simulink model "TST_CrCtl_ShOff"  (R2016b)
settings: Solver=FixedStepDiscrete  StartTime=0.0  StopTime=simTime  FixedStep=sampleTime  RelTol=1e-3
values from neighbouring files (symbols this model uses):
  testCase = 1    [initTST_CrCtl_ShOff_001.m]    (also in initTST_CrCtl_ShOff_002.m = 2; initTST_CrCtl_ShOff_003.m = 3)
libraries: simulink x31, UnitTest_Lib x15
(part 1 of 2)
settings Model: Creator=guanxiaoxing  LastModifiedBy=guanxiaoxing
settings DebuggingCC: SignalRangeChecking=error

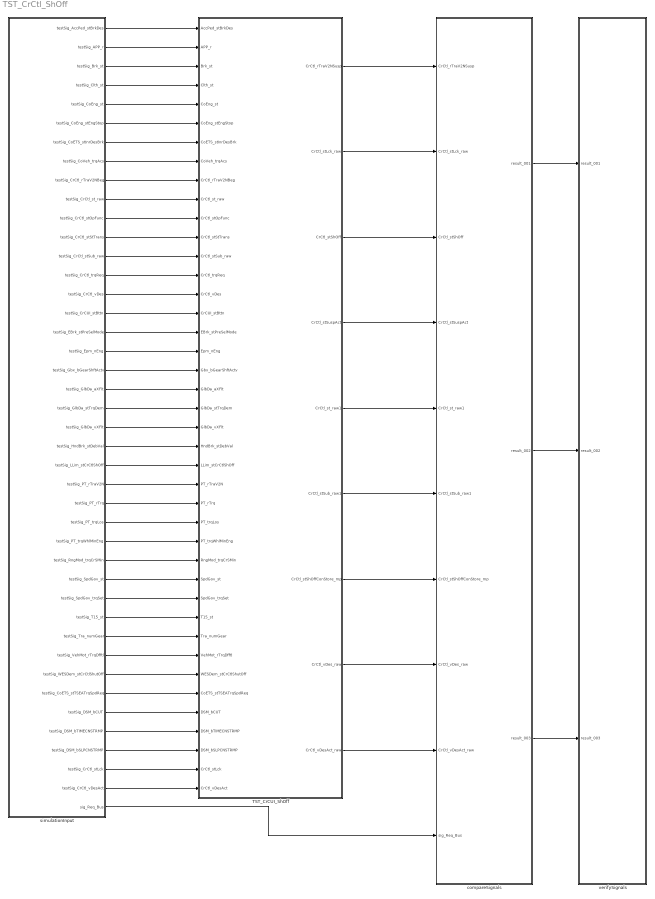
== system TST_CrCtl_ShOff ==
  TST_CrCUI_ShOff : Subsystem
  compareSignals : Subsystem
  simulationInput : Subsystem
  verifySignals : Subsystem
  wires:
  simulationInput/1(testSig_AccPed_stBrkDes) -> TST_CrCUI_ShOff/1(AccPed_stBrkDes)
  simulationInput/2(testSig_APP_r) -> TST_CrCUI_ShOff/2(APP_r)
  simulationInput/3(testSig_Brk_st) -> TST_CrCUI_ShOff/3(Brk_st)
  simulationInput/4(testSig_Clth_st) -> TST_CrCUI_ShOff/4(Clth_st)
  simulationInput/5(testSig_CoEng_st) -> TST_CrCUI_ShOff/5(CoEng_st)
  simulationInput/6(testSig_CoEng_stEngStop) -> TST_CrCUI_ShOff/6(CoEng_stEngStop)
  simulationInput/7(testSig_CoETS_stInrDesBrk) -> TST_CrCUI_ShOff/7(CoETS_stInrDesBrk)
  simulationInput/8(testSig_CoVeh_trqAcs) -> TST_CrCUI_ShOff/8(CoVeh_trqAcs)
  simulationInput/9(testSig_CrCtl_rTraV2NBeg) -> TST_CrCUI_ShOff/9(CrCtl_rTraV2NBeg)
  simulationInput/10(testSig_CrCtl_st_raw) -> TST_CrCUI_ShOff/10(CrCtl_st_raw)
  simulationInput/11(testSig_CrCtl_stOpFunc) -> TST_CrCUI_ShOff/11(CrCtl_stOpFunc)
  simulationInput/12(testSig_CrCtl_stStTrans) -> TST_CrCUI_ShOff/12(CrCtl_stStTrans)
  simulationInput/13(testSig_CrCtl_stSub_raw) -> TST_CrCUI_ShOff/13(CrCtl_stSub_raw)
  simulationInput/14(testSig_CrCtl_trqReq) -> TST_CrCUI_ShOff/14(CrCtl_trqReq)
  simulationInput/15(testSig_CrCtl_vDes) -> TST_CrCUI_ShOff/15(CrCtl_vDes)
  simulationInput/16(testSig_CrCUI_stBttn) -> TST_CrCUI_ShOff/16(CrCUI_stBttn)
  simulationInput/17(testSig_EBrk_stPreSelMode) -> TST_CrCUI_ShOff/17(EBrk_stPreSelMode)
  simulationInput/18(testSig_Epm_nEng) -> TST_CrCUI_ShOff/18(Epm_nEng)
  simulationInput/19(testSig_Gbx_bGearShftActv) -> TST_CrCUI_ShOff/19(Gbx_bGearShftActv)
  simulationInput/20(testSig_GlbDa_aXFlt) -> TST_CrCUI_ShOff/20(GlbDa_aXFlt)
  simulationInput/21(testSig_GlbDa_stTrqDem) -> TST_CrCUI_ShOff/21(GlbDa_stTrqDem)
  simulationInput/22(testSig_GlbDa_vXFlt) -> TST_CrCUI_ShOff/22(GlbDa_vXFlt)
  simulationInput/23(testSig_HndBrk_stDebVal) -> TST_CrCUI_ShOff/23(HndBrk_stDebVal)
  simulationInput/24(testSig_LLim_stCrCtlShOff) -> TST_CrCUI_ShOff/24(LLim_stCrCtlShOff)
  simulationInput/25(testSig_PT_rTraV2N) -> TST_CrCUI_ShOff/25(PT_rTraV2N)
  simulationInput/26(testSig_PT_rTrq) -> TST_CrCUI_ShOff/26(PT_rTrq)
  simulationInput/27(testSig_PT_trqLos) -> TST_CrCUI_ShOff/27(PT_trqLos)
  simulationInput/28(testSig_PT_trqWhlMinEng) -> TST_CrCUI_ShOff/28(PT_trqWhlMinEng)
  simulationInput/29(testSig_RngMod_trqCrSMin) -> TST_CrCUI_ShOff/29(RngMod_trqCrSMin)
  simulationInput/30(testSig_SpdGov_st) -> TST_CrCUI_ShOff/30(SpdGov_st)
  simulationInput/31(testSig_SpdGov_trqSet) -> TST_CrCUI_ShOff/31(SpdGov_trqSet)
  simulationInput/32(testSig_T15_st) -> TST_CrCUI_ShOff/32(T15_st)
  simulationInput/33(testSig_Tra_numGear) -> TST_CrCUI_ShOff/33(Tra_numGear)
  simulationInput/34(testSig_VehMot_rTrqDfftl) -> TST_CrCUI_ShOff/34(VehMot_rTrqDfftl)
  simulationInput/35(testSig_WESDem_stCrCtlShutOff) -> TST_CrCUI_ShOff/35(WESDem_stCrCtlShutOff)
  simulationInput/36(testSig_CoETS_stTSEATrqSpdReq) -> TST_CrCUI_ShOff/36(CoETS_stTSEATrqSpdReq)
  simulationInput/37(testSig_DSM_bCUT) -> TST_CrCUI_ShOff/37(DSM_bCUT)
  simulationInput/38(testSig_DSM_bTIMECNSTRMP) -> TST_CrCUI_ShOff/38(DSM_bTIMECNSTRMP)
  simulationInput/39(testSig_DSM_bSLPCNSTRMP) -> TST_CrCUI_ShOff/39(DSM_bSLPCNSTRMP)
  simulationInput/40(testSig_CrCtl_stLck) -> TST_CrCUI_ShOff/40(CrCtl_stLck)
  simulationInput/41(testSig_CrCtl_vDesAct) -> TST_CrCUI_ShOff/41(CrCtl_vDesAct)
  TST_CrCUI_ShOff/1(CrCtl_rTraV2NSusp) -> compareSignals/1(CrCtl_rTraV2NSusp)
  TST_CrCUI_ShOff/2(CrCtl_stLck_raw) -> compareSignals/2(CrCtl_stLck_raw)
  TST_CrCUI_ShOff/3(CrCtl_stShOff) -> compareSignals/3(CrCtl_stShOff)
  TST_CrCUI_ShOff/4(CrCtl_stSuspAct) -> compareSignals/4(CrCtl_stSuspAct)
  TST_CrCUI_ShOff/5(CrCtl_st_raw1) -> compareSignals/5(CrCtl_st_raw1)
  TST_CrCUI_ShOff/6(CrCtl_stSub_raw1) -> compareSignals/6(CrCtl_stSub_raw1)
  TST_CrCUI_ShOff/7(CrCtl_stShOffConStore_mp) -> compareSignals/7(CrCtl_stShOffConStore_mp)
  TST_CrCUI_ShOff/8(CrCtl_vDes_raw) -> compareSignals/8(CrCtl_vDes_raw)
  TST_CrCUI_ShOff/9(CrCtl_vDesAct_raw) -> compareSignals/9(CrCtl_vDesAct_raw)
  simulationInput/42(sig_Req_Bus) -> compareSignals/10(sig_Req_Bus)
  compareSignals/1(result_001) -> verifySignals/1(result_001)
  compareSignals/2(result_002) -> verifySignals/2(result_002)
  compareSignals/3(result_003) -> verifySignals/3(result_003)

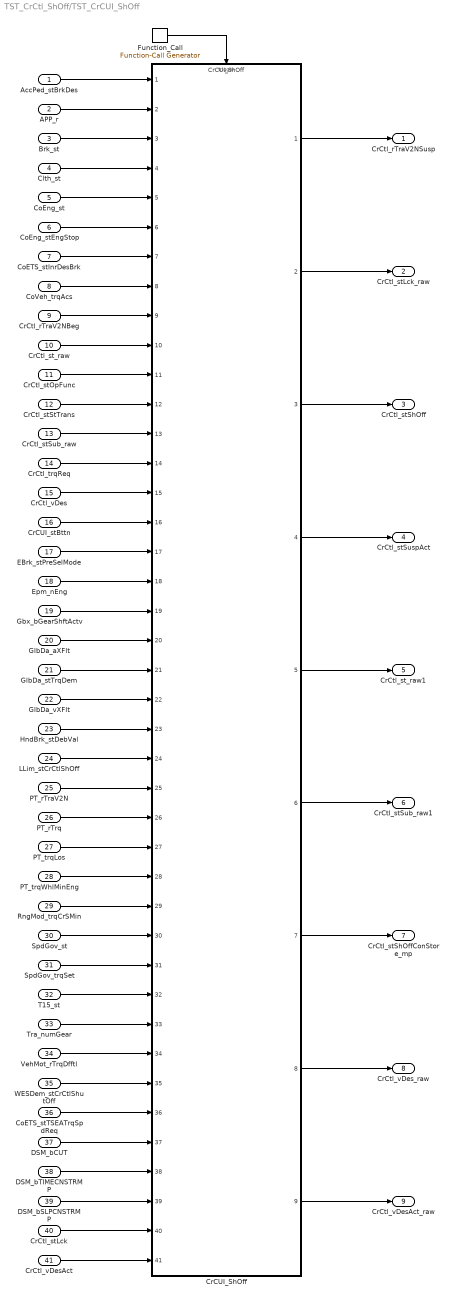
== system TST_CrCtl_ShOff/TST_CrCUI_ShOff ==
  AccPed_stBrkDes : Inport
  APP_r : Inport  Port=2
  Brk_st : Inport  Port=3
  Clth_st : Inport  Port=4
  CoEng_st : Inport  Port=5
  CoEng_stEngStop : Inport  Port=6
  CoETS_stInrDesBrk : Inport  Port=7
  CoVeh_trqAcs : Inport  Port=8
  CrCtl_rTraV2NBeg : Inport  Port=9
  CrCtl_st_raw : Inport  Port=10
  CrCtl_stOpFunc : Inport  Port=11
  CrCtl_stStTrans : Inport  Port=12
  CrCtl_stSub_raw : Inport  Port=13
  CrCtl_trqReq : Inport  Port=14
  CrCtl_vDes : Inport  Port=15
  CrCUI_stBttn : Inport  Port=16
  EBrk_stPreSelMode : Inport  Port=17
  Epm_nEng : Inport  Port=18
  Gbx_bGearShftActv : Inport  Port=19
  GlbDa_aXFlt : Inport  Port=20
  GlbDa_stTrqDem : Inport  Port=21
  GlbDa_vXFlt : Inport  Port=22
  HndBrk_stDebVal : Inport  Port=23
  LLim_stCrCtlShOff : Inport  Port=24
  PT_rTraV2N : Inport  Port=25
  PT_rTrq : Inport  Port=26
  PT_trqLos : Inport  Port=27
  PT_trqWhlMinEng : Inport  Port=28
  RngMod_trqCrSMin : Inport  Port=29
  SpdGov_st : Inport  Port=30
  SpdGov_trqSet : Inport  Port=31
  T15_st : Inport  Port=32
  Tra_numGear : Inport  Port=33
  VehMot_rTrqDfftl : Inport  Port=34
  WESDem_stCrCtlShutOff : Inport  Port=35
  CoETS_stTSEATrqSpdReq : Inport  Port=36
  DSM_bCUT : Inport  Port=37
  DSM_bTIMECNSTRMP : Inport  Port=38
  DSM_bSLPCNSTRMP : Inport  Port=39
  CrCtl_stLck : Inport  Port=40
  CrCtl_vDesAct : Inport  Port=41
  CrCUI_ShOff : ModelReference  ModelNameDialog=CrCUI_ShOff  SimulationMode=Normal  ModelReferenceVersion=1.124  TriggerPortName=function  TriggerPortTriggerType=function-call  TriggerPortStatesWhenEnabling=held
  Function_Call : simulink/Ports & Subsystems/Function-Call Generator  sample_time=sampleTime  numberOfIterations=1
  CrCtl_rTraV2NSusp : Outport
  CrCtl_stLck_raw : Outport  Port=2
  CrCtl_stShOff : Outport  Port=3
  CrCtl_stSuspAct : Outport  Port=4
  CrCtl_st_raw1 : Outport  Port=5
  CrCtl_stSub_raw1 : Outport  Port=6
  CrCtl_stShOffConStore_mp : Outport  Port=7
  CrCtl_vDes_raw : Outport  Port=8
  CrCtl_vDesAct_raw : Outport  Port=9
  wires:
  Function_Call/1 -> CrCUI_ShOff/Trigger
  AccPed_stBrkDes/1 -> CrCUI_ShOff/1
  APP_r/1 -> CrCUI_ShOff/2
  Brk_st/1 -> CrCUI_ShOff/3
  Clth_st/1 -> CrCUI_ShOff/4
  CoEng_st/1 -> CrCUI_ShOff/5
  CoEng_stEngStop/1 -> CrCUI_ShOff/6
  CoETS_stInrDesBrk/1 -> CrCUI_ShOff/7
  CoVeh_trqAcs/1 -> CrCUI_ShOff/8
  CrCtl_rTraV2NBeg/1 -> CrCUI_ShOff/9
  CrCtl_st_raw/1 -> CrCUI_ShOff/10
  CrCtl_stOpFunc/1 -> CrCUI_ShOff/11
  CrCtl_stStTrans/1 -> CrCUI_ShOff/12
  CrCtl_stSub_raw/1 -> CrCUI_ShOff/13
  CrCtl_trqReq/1 -> CrCUI_ShOff/14
  CrCtl_vDes/1 -> CrCUI_ShOff/15
  CrCUI_stBttn/1 -> CrCUI_ShOff/16
  EBrk_stPreSelMode/1 -> CrCUI_ShOff/17
  Epm_nEng/1 -> CrCUI_ShOff/18
  Gbx_bGearShftActv/1 -> CrCUI_ShOff/19
  GlbDa_aXFlt/1 -> CrCUI_ShOff/20
  GlbDa_stTrqDem/1 -> CrCUI_ShOff/21
  GlbDa_vXFlt/1 -> CrCUI_ShOff/22
  HndBrk_stDebVal/1 -> CrCUI_ShOff/23
  LLim_stCrCtlShOff/1 -> CrCUI_ShOff/24
  PT_rTraV2N/1 -> CrCUI_ShOff/25
  PT_rTrq/1 -> CrCUI_ShOff/26
  PT_trqLos/1 -> CrCUI_ShOff/27
  PT_trqWhlMinEng/1 -> CrCUI_ShOff/28
  RngMod_trqCrSMin/1 -> CrCUI_ShOff/29
  SpdGov_st/1 -> CrCUI_ShOff/30
  SpdGov_trqSet/1 -> CrCUI_ShOff/31
  T15_st/1 -> CrCUI_ShOff/32
  Tra_numGear/1 -> CrCUI_ShOff/33
  VehMot_rTrqDfftl/1 -> CrCUI_ShOff/34
  WESDem_stCrCtlShutOff/1 -> CrCUI_ShOff/35
  CoETS_stTSEATrqSpdReq/1 -> CrCUI_ShOff/36
  DSM_bCUT/1 -> CrCUI_ShOff/37
  DSM_bTIMECNSTRMP/1 -> CrCUI_ShOff/38
  DSM_bSLPCNSTRMP/1 -> CrCUI_ShOff/39
  CrCtl_stLck/1 -> CrCUI_ShOff/40
  CrCtl_vDesAct/1 -> CrCUI_ShOff/41
  CrCUI_ShOff/1 -> CrCtl_rTraV2NSusp/1
  CrCUI_ShOff/2 -> CrCtl_stLck_raw/1
  CrCUI_ShOff/3 -> CrCtl_stShOff/1
  CrCUI_ShOff/4 -> CrCtl_stSuspAct/1
  CrCUI_ShOff/5 -> CrCtl_st_raw1/1
  CrCUI_ShOff/6 -> CrCtl_stSub_raw1/1
  CrCUI_ShOff/7 -> CrCtl_stShOffConStore_mp/1
  CrCUI_ShOff/8 -> CrCtl_vDes_raw/1
  CrCUI_ShOff/9 -> CrCtl_vDesAct_raw/1

== system TST_CrCtl_ShOff/compareSignals ==
  CrCtl_rTraV2NSusp : Inport
  CrCtl_stLck_raw : Inport  Port=2
  CrCtl_stShOff : Inport  Port=3
  CrCtl_stSuspAct : Inport  Port=4
  CrCtl_st_raw1 : Inport  Port=5
  CrCtl_stSub_raw1 : Inport  Port=6
  CrCtl_stShOffConStore_mp : Inport  Port=7
  CrCtl_vDes_raw : Inport  Port=8
  CrCtl_vDesAct_raw : Inport  Port=9
  sig_Req_Bus : Inport  Port=10
  BC : BusCreator  Inputs=9
  CTC_001 : simulink/Logic and Bit Operations/Compare To Constant  relop===  const=1  OutDataTypeStr=boolean
  CTC_002 : simulink/Logic and Bit Operations/Compare To Constant  relop===  const=2  OutDataTypeStr=boolean
  CTC_003 : simulink/Logic and Bit Operations/Compare To Constant  relop===  const=3  OutDataTypeStr=boolean
  Requirement_001 : Subsystem
  Requirement_002 : Subsystem
  Requirement_003 : Subsystem
  TC_001 : Constant  Value=testCase
  TC_002 : Constant  Value=testCase
  TC_003 : Constant  Value=testCase
  result_001 : Outport
  result_002 : Outport  Port=2
  result_003 : Outport  Port=3
  wires:
  CrCtl_rTraV2NSusp/1 -> BC/1  "CrCtl_rTraV2NSusp"
  CrCtl_stLck_raw/1 -> BC/2  "CrCtl_stLck_raw"
  CrCtl_stShOff/1 -> BC/3  "CrCtl_stShOff"
  CrCtl_stSuspAct/1 -> BC/4  "CrCtl_stSuspAct"
  CrCtl_st_raw1/1 -> BC/5  "CrCtl_st_raw1"
  CrCtl_stSub_raw1/1 -> BC/6  "CrCtl_stSub_raw1"
  CrCtl_stShOffConStore_mp/1 -> BC/7  "CrCtl_stShOffConStore_mp"
  CrCtl_vDes_raw/1 -> BC/8  "CrCtl_vDes_raw"
  CrCtl_vDesAct_raw/1 -> BC/9  "CrCtl_vDesAct_raw"
  TC_001/1 -> CTC_001/1
  CTC_001/1 -> Requirement_001/Enable
  sig_Req_Bus/1 -> Requirement_001/2(sig_Req_Bus), Requirement_002/2(sig_Req_Bus), Requirement_003/2(sig_Req_Bus)
  BC/1 -> Requirement_002/1(sig_Result_Bus), Requirement_003/1(sig_Result_Bus), Requirement_001/1(sig_Result_Bus)
  Requirement_001/1(result) -> result_001/1
  TC_002/1 -> CTC_002/1
  CTC_002/1 -> Requirement_002/Enable
  Requirement_002/1(result) -> result_002/1
  TC_003/1 -> CTC_003/1
  CTC_003/1 -> Requirement_003/Enable
  Requirement_003/1(result) -> result_003/1

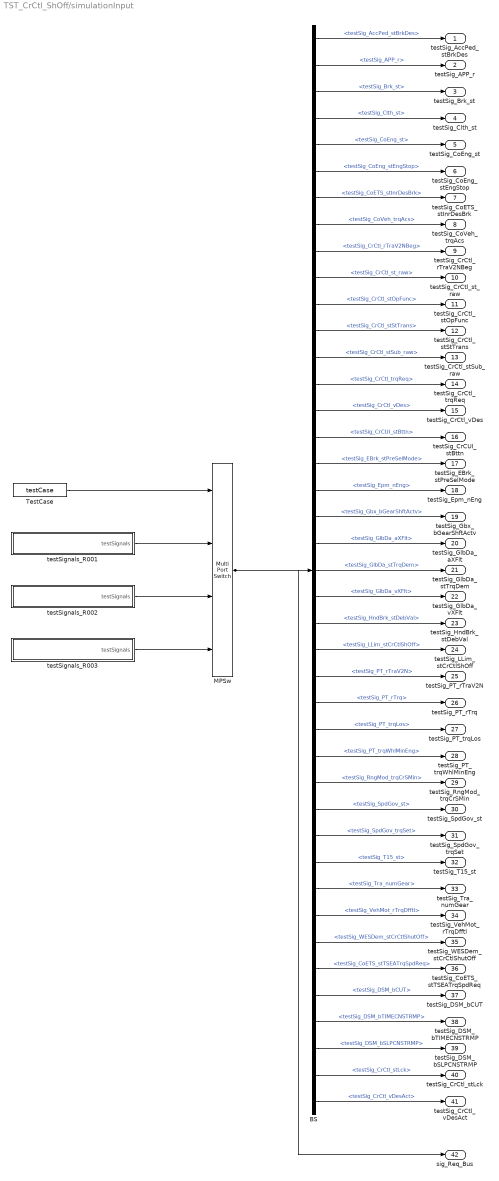
== system TST_CrCtl_ShOff/simulationInput ==
  BS : BusSelector  OutputSignals=testSig_AccPed_stBrkDes,testSig_APP_r,testSig_Brk_st,testSig_Clth_st,testSig_CoEng_st,testSig_CoEng_stEngStop,testSig_CoETS_stInrDesBrk,testSig_CoVeh_trqAcs,testSig_CrCtl_rTraV2NBeg,testSig_CrCtl_st_raw,testSig_CrCtl_stOpFunc,testSig_CrCtl_stStTrans,testSig_CrCtl_stSub_raw,testSig_CrCtl_trqReq,testSig_CrCtl_vDes,testSig_CrCUI_stBttn,testSig_EBrk_stPreSelMode,testSig_Epm_nEng,testSig_Gbx_bGearShftActv,testSig_GlbDa_aXFlt,testSig_GlbDa_stTrqDem,testSig_GlbDa_vXFlt,testSig_HndBrk_stDebVal,testSig_LLim_stCrCtlShOff,testSig_PT_rTraV2N,testSig_PT_rTrq,testSig_PT_trqLos,testSig_PT_trqWhlMinEng,testSig_RngMod_trqCrSMin,testSig_SpdGov_st,testSig_SpdGov_trqSet,testSig_T15_st,testSig_Tra_numGear,testSig_VehMot_rTrqDfftl,testSig_WESDem_stCrCtlShutOff,testSig_CoETS_stTSEATrqSpdReq,testSig_DSM_bCUT,testSig_DSM_bTIMECNSTRMP,testSig_DSM_bSLPCNSTRMP,testSig_CrCtl_stLck,testSig_CrCtl_vDesAct
  MPSw : MultiPortSwitch  SaturateOnIntegerOverflow=on  InputSameDT=on
  TestCase : Constant  Value=testCase
  testSignals_R001 : Subsystem
  testSignals_R002 : Subsystem
  testSignals_R003 : Subsystem
  testSig_AccPed_stBrkDes : Outport
  testSig_APP_r : Outport  Port=2
  testSig_Brk_st : Outport  Port=3
  testSig_Clth_st : Outport  Port=4
  testSig_CoEng_st : Outport  Port=5
  testSig_CoEng_stEngStop : Outport  Port=6
  testSig_CoETS_stInrDesBrk : Outport  Port=7
  testSig_CoVeh_trqAcs : Outport  Port=8
  testSig_CrCtl_rTraV2NBeg : Outport  Port=9
  testSig_CrCtl_st_raw : Outport  Port=10
  testSig_CrCtl_stOpFunc : Outport  Port=11
  testSig_CrCtl_stStTrans : Outport  Port=12
  testSig_CrCtl_stSub_raw : Outport  Port=13
  testSig_CrCtl_trqReq : Outport  Port=14
  testSig_CrCtl_vDes : Outport  Port=15
  testSig_CrCUI_stBttn : Outport  Port=16
  testSig_EBrk_stPreSelMode : Outport  Port=17
  testSig_Epm_nEng : Outport  Port=18
  testSig_Gbx_bGearShftActv : Outport  Port=19
  testSig_GlbDa_aXFlt : Outport  Port=20
  testSig_GlbDa_stTrqDem : Outport  Port=21
  testSig_GlbDa_vXFlt : Outport  Port=22
  testSig_HndBrk_stDebVal : Outport  Port=23
  testSig_LLim_stCrCtlShOff : Outport  Port=24
  testSig_PT_rTraV2N : Outport  Port=25
  testSig_PT_rTrq : Outport  Port=26
  testSig_PT_trqLos : Outport  Port=27
  testSig_PT_trqWhlMinEng : Outport  Port=28
  testSig_RngMod_trqCrSMin : Outport  Port=29
  testSig_SpdGov_st : Outport  Port=30
  testSig_SpdGov_trqSet : Outport  Port=31
  testSig_T15_st : Outport  Port=32
  testSig_Tra_numGear : Outport  Port=33
  testSig_VehMot_rTrqDfftl : Outport  Port=34
  testSig_WESDem_stCrCtlShutOff : Outport  Port=35
  testSig_CoETS_stTSEATrqSpdReq : Outport  Port=36
  testSig_DSM_bCUT : Outport  Port=37
  testSig_DSM_bTIMECNSTRMP : Outport  Port=38
  testSig_DSM_bSLPCNSTRMP : Outport  Port=39
  testSig_CrCtl_stLck : Outport  Port=40
  testSig_CrCtl_vDesAct : Outport  Port=41
  sig_Req_Bus : Outport  Port=42
  wires:
  BS/1 -> testSig_AccPed_stBrkDes/1  "<testSig_AccPed_stBrkDes>"
  BS/2 -> testSig_APP_r/1  "<testSig_APP_r>"
  BS/3 -> testSig_Brk_st/1  "<testSig_Brk_st>"
  BS/4 -> testSig_Clth_st/1  "<testSig_Clth_st>"
  BS/5 -> testSig_CoEng_st/1  "<testSig_CoEng_st>"
  BS/6 -> testSig_CoEng_stEngStop/1  "<testSig_CoEng_stEngStop>"
  BS/7 -> testSig_CoETS_stInrDesBrk/1  "<testSig_CoETS_stInrDesBrk>"
  BS/8 -> testSig_CoVeh_trqAcs/1  "<testSig_CoVeh_trqAcs>"
  BS/9 -> testSig_CrCtl_rTraV2NBeg/1  "<testSig_CrCtl_rTraV2NBeg>"
  BS/10 -> testSig_CrCtl_st_raw/1  "<testSig_CrCtl_st_raw>"
  BS/11 -> testSig_CrCtl_stOpFunc/1  "<testSig_CrCtl_stOpFunc>"
  BS/12 -> testSig_CrCtl_stStTrans/1  "<testSig_CrCtl_stStTrans>"
  BS/13 -> testSig_CrCtl_stSub_raw/1  "<testSig_CrCtl_stSub_raw>"
  BS/14 -> testSig_CrCtl_trqReq/1  "<testSig_CrCtl_trqReq>"
  BS/15 -> testSig_CrCtl_vDes/1  "<testSig_CrCtl_vDes>"
  BS/16 -> testSig_CrCUI_stBttn/1  "<testSig_CrCUI_stBttn>"
  BS/17 -> testSig_EBrk_stPreSelMode/1  "<testSig_EBrk_stPreSelMode>"
  BS/18 -> testSig_Epm_nEng/1  "<testSig_Epm_nEng>"
  BS/19 -> testSig_Gbx_bGearShftActv/1  "<testSig_Gbx_bGearShftActv>"
  BS/20 -> testSig_GlbDa_aXFlt/1  "<testSig_GlbDa_aXFlt>"
  BS/21 -> testSig_GlbDa_stTrqDem/1  "<testSig_GlbDa_stTrqDem>"
  BS/22 -> testSig_GlbDa_vXFlt/1  "<testSig_GlbDa_vXFlt>"
  BS/23 -> testSig_HndBrk_stDebVal/1  "<testSig_HndBrk_stDebVal>"
  BS/24 -> testSig_LLim_stCrCtlShOff/1  "<testSig_LLim_stCrCtlShOff>"
  BS/25 -> testSig_PT_rTraV2N/1  "<testSig_PT_rTraV2N>"
  BS/26 -> testSig_PT_rTrq/1  "<testSig_PT_rTrq>"
  BS/27 -> testSig_PT_trqLos/1  "<testSig_PT_trqLos>"
  BS/28 -> testSig_PT_trqWhlMinEng/1  "<testSig_PT_trqWhlMinEng>"
  BS/29 -> testSig_RngMod_trqCrSMin/1  "<testSig_RngMod_trqCrSMin>"
  BS/30 -> testSig_SpdGov_st/1  "<testSig_SpdGov_st>"
  BS/31 -> testSig_SpdGov_trqSet/1  "<testSig_SpdGov_trqSet>"
  BS/32 -> testSig_T15_st/1  "<testSig_T15_st>"
  BS/33 -> testSig_Tra_numGear/1  "<testSig_Tra_numGear>"
  BS/34 -> testSig_VehMot_rTrqDfftl/1  "<testSig_VehMot_rTrqDfftl>"
  BS/35 -> testSig_WESDem_stCrCtlShutOff/1  "<testSig_WESDem_stCrCtlShutOff>"
  BS/36 -> testSig_CoETS_stTSEATrqSpdReq/1  "<testSig_CoETS_stTSEATrqSpdReq>"
  BS/37 -> testSig_DSM_bCUT/1  "<testSig_DSM_bCUT>"
  BS/38 -> testSig_DSM_bTIMECNSTRMP/1  "<testSig_DSM_bTIMECNSTRMP>"
  BS/39 -> testSig_DSM_bSLPCNSTRMP/1  "<testSig_DSM_bSLPCNSTRMP>"
  BS/40 -> testSig_CrCtl_stLck/1  "<testSig_CrCtl_stLck>"
  BS/41 -> testSig_CrCtl_vDesAct/1  "<testSig_CrCtl_vDesAct>"
  MPSw/1 -> BS/1, sig_Req_Bus/1
  TestCase/1 -> MPSw/1
  testSignals_R001/1(testSignals) -> MPSw/2
  testSignals_R002/1(testSignals) -> MPSw/3
  testSignals_R003/1(testSignals) -> MPSw/4

== system TST_CrCtl_ShOff/verifySignals ==
  result_001 : Inport
  result_002 : Inport  Port=2
  result_003 : Inport  Port=3
  Assertion_001 : Assertion  Enabled=off
  Assertion_002 : Assertion  Enabled=off
  Assertion_003 : Assertion  Enabled=off
  wires:
  result_001/1 -> Assertion_001/1
  result_002/1 -> Assertion_002/1
  result_003/1 -> Assertion_003/1

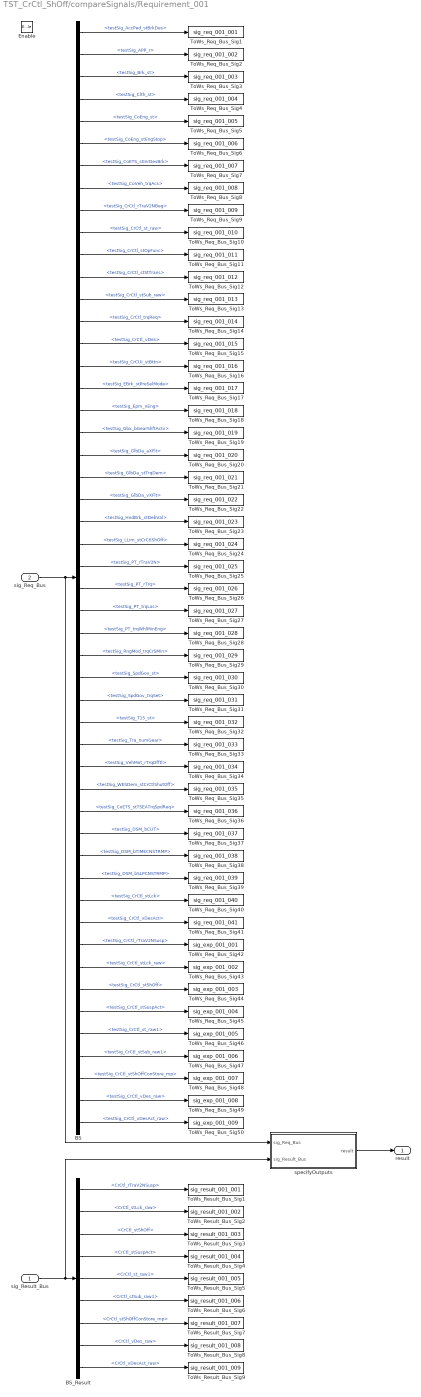
== system TST_CrCtl_ShOff/compareSignals/Requirement_001 ==
  sig_Result_Bus : Inport
  sig_Req_Bus : Inport  Port=2
  Enable : EnablePort
  BS : BusSelector  OutputSignals=testSig_AccPed_stBrkDes,testSig_APP_r,testSig_Brk_st,testSig_Clth_st,testSig_CoEng_st,testSig_CoEng_stEngStop,testSig_CoETS_stInrDesBrk,testSig_CoVeh_trqAcs,testSig_CrCtl_rTraV2NBeg,testSig_CrCtl_st_raw,testSig_CrCtl_stOpFunc,testSig_CrCtl_stStTrans,testSig_CrCtl_stSub_raw,testSig_CrCtl_trqReq,testSig_CrCtl_vDes,testSig_CrCUI_stBttn,testSig_EBrk_stPreSelMode,testSig_Epm_nEng,testSig_Gbx_bGearShftActv,testSig_GlbDa_aXFlt,testSig_GlbDa_stTrqDem,testSig_GlbDa_vXFlt,testSig_HndBrk_stDebVal,testSig_LLim_stCrCtlShOff,testSig_PT_rTraV2N,testSig_PT_rTrq,testSig_PT_trqLos,testSig_PT_trqWhlMinEng,testSig_RngMod_trqCrSMin,testSig_SpdGov_st,testSig_SpdGov_trqSet,testSig_T15_st,testSig_Tra_numGear,testSig_VehMot_rTrqDfftl,testSig_WESDem_stCrCtlShutOff,testSig_CoETS_stTSEATrqSpdReq,testSig_DSM_bCUT,testSig_DSM_bTIMECNSTRMP,testSig_DSM_bSLPCNSTRMP,testSig_CrCtl_stLck,testSig_CrCtl_vDesAct,testSig_CrCtl_rTraV2NSusp,testSig_CrCtl_stLck_raw,testSig_CrCtl_stShOff,testSig_CrCtl_stSuspAct,testSig_CrCtl_st_raw1,testSig_CrCtl_stSub_raw1,testSig_CrCtl_stShOffConStore_mp,testSig_CrCtl_vDes_raw,testSig_CrCtl_vDesAct_raw
  BS_Result : BusSelector  OutputSignals=CrCtl_rTraV2NSusp,CrCtl_stLck_raw,CrCtl_stShOff,CrCtl_stSuspAct,CrCtl_st_raw1,CrCtl_stSub_raw1,CrCtl_stShOffConStore_mp,CrCtl_vDes_raw,CrCtl_vDesAct_raw
  ToWs_Req_Bus_Sig1 : ToWorkspace  VariableName=sig_req_001_001  SaveFormat=Structure With Time
  ToWs_Req_Bus_Sig10 : ToWorkspace  VariableName=sig_req_001_010  SaveFormat=Structure With Time
  ToWs_Req_Bus_Sig11 : ToWorkspace  VariableName=sig_req_001_011  SaveFormat=Structure With Time
  ToWs_Req_Bus_Sig12 : ToWorkspace  VariableName=sig_req_001_012  SaveFormat=Structure With Time
  ToWs_Req_Bus_Sig13 : ToWorkspace  VariableName=sig_req_001_013  SaveFormat=Structure With Time
  ToWs_Req_Bus_Sig14 : ToWorkspace  VariableName=sig_req_001_014  SaveFormat=Structure With Time
  ToWs_Req_Bus_Sig15 : ToWorkspace  VariableName=sig_req_001_015  SaveFormat=Structure With Time
  ToWs_Req_Bus_Sig16 : ToWorkspace  VariableName=sig_req_001_016  SaveFormat=Structure With Time
  ToWs_Req_Bus_Sig17 : ToWorkspace  VariableName=sig_req_001_017  SaveFormat=Structure With Time
  ToWs_Req_Bus_Sig18 : ToWorkspace  VariableName=sig_req_001_018  SaveFormat=Structure With Time
  ToWs_Req_Bus_Sig19 : ToWorkspace  VariableName=sig_req_001_019  SaveFormat=Structure With Time
  ToWs_Req_Bus_Sig2 : ToWorkspace  VariableName=sig_req_001_002  SaveFormat=Structure With Time
  ToWs_Req_Bus_Sig20 : ToWorkspace  VariableName=sig_req_001_020  SaveFormat=Structure With Time
  ToWs_Req_Bus_Sig21 : ToWorkspace  VariableName=sig_req_001_021  SaveFormat=Structure With Time
  ToWs_Req_Bus_Sig22 : ToWorkspace  VariableName=sig_req_001_022  SaveFormat=Structure With Time
  ToWs_Req_Bus_Sig23 : ToWorkspace  VariableName=sig_req_001_023  SaveFormat=Structure With Time
  ToWs_Req_Bus_Sig24 : ToWorkspace  VariableName=sig_req_001_024  SaveFormat=Structure With Time
  ToWs_Req_Bus_Sig25 : ToWorkspace  VariableName=sig_req_001_025  SaveFormat=Structure With Time
  ToWs_Req_Bus_Sig26 : ToWorkspace  VariableName=sig_req_001_026  SaveFormat=Structure With Time
  ToWs_Req_Bus_Sig27 : ToWorkspace  VariableName=sig_req_001_027  SaveFormat=Structure With Time
  ToWs_Req_Bus_Sig28 : ToWorkspace  VariableName=sig_req_001_028  SaveFormat=Structure With Time
  ToWs_Req_Bus_Sig29 : ToWorkspace  VariableName=sig_req_001_029  SaveFormat=Structure With Time
  ToWs_Req_Bus_Sig3 : ToWorkspace  VariableName=sig_req_001_003  SaveFormat=Structure With Time
  ToWs_Req_Bus_Sig30 : ToWorkspace  VariableName=sig_req_001_030  SaveFormat=Structure With Time
  ToWs_Req_Bus_Sig31 : ToWorkspace  VariableName=sig_req_001_031  SaveFormat=Structure With Time
  ToWs_Req_Bus_Sig32 : ToWorkspace  VariableName=sig_req_001_032  SaveFormat=Structure With Time
  ToWs_Req_Bus_Sig33 : ToWorkspace  VariableName=sig_req_001_033  SaveFormat=Structure With Time
  ToWs_Req_Bus_Sig34 : ToWorkspace  VariableName=sig_req_001_034  SaveFormat=Structure With Time
  ToWs_Req_Bus_Sig35 : ToWorkspace  VariableName=sig_req_001_035  SaveFormat=Structure With Time
  ToWs_Req_Bus_Sig36 : ToWorkspace  VariableName=sig_req_001_036  SaveFormat=Structure With Time
  ToWs_Req_Bus_Sig37 : ToWorkspace  VariableName=sig_req_001_037  SaveFormat=Structure With Time
  ToWs_Req_Bus_Sig38 : ToWorkspace  VariableName=sig_req_001_038  SaveFormat=Structure With Time
  ToWs_Req_Bus_Sig39 : ToWorkspace  VariableName=sig_req_001_039  SaveFormat=Structure With Time
  ToWs_Req_Bus_Sig4 : ToWorkspace  VariableName=sig_req_001_004  SaveFormat=Structure With Time
  ToWs_Req_Bus_Sig40 : ToWorkspace  VariableName=sig_req_001_040  SaveFormat=Structure With Time
  ToWs_Req_Bus_Sig41 : ToWorkspace  VariableName=sig_req_001_041  SaveFormat=Structure With Time
  ToWs_Req_Bus_Sig42 : ToWorkspace  VariableName=sig_exp_001_001  SaveFormat=Structure With Time
  ToWs_Req_Bus_Sig43 : ToWorkspace  VariableName=sig_exp_001_002  SaveFormat=Structure With Time
  ToWs_Req_Bus_Sig44 : ToWorkspace  VariableName=sig_exp_001_003  SaveFormat=Structure With Time
  ToWs_Req_Bus_Sig45 : ToWorkspace  VariableName=sig_exp_001_004  SaveFormat=Structure With Time
  ToWs_Req_Bus_Sig46 : ToWorkspace  VariableName=sig_exp_001_005  SaveFormat=Structure With Time
  ToWs_Req_Bus_Sig47 : ToWorkspace  VariableName=sig_exp_001_006  SaveFormat=Structure With Time
  ToWs_Req_Bus_Sig48 : ToWorkspace  VariableName=sig_exp_001_007  SaveFormat=Structure With Time
  ToWs_Req_Bus_Sig49 : ToWorkspace  VariableName=sig_exp_001_008  SaveFormat=Structure With Time
  ToWs_Req_Bus_Sig5 : ToWorkspace  VariableName=sig_req_001_005  SaveFormat=Structure With Time
  ToWs_Req_Bus_Sig50 : ToWorkspace  VariableName=sig_exp_001_009  SaveFormat=Structure With Time
  ToWs_Req_Bus_Sig6 : ToWorkspace  VariableName=sig_req_001_006  SaveFormat=Structure With Time
  ToWs_Req_Bus_Sig7 : ToWorkspace  VariableName=sig_req_001_007  SaveFormat=Structure With Time
  ToWs_Req_Bus_Sig8 : ToWorkspace  VariableName=sig_req_001_008  SaveFormat=Structure With Time
  ToWs_Req_Bus_Sig9 : ToWorkspace  VariableName=sig_req_001_009  SaveFormat=Structure With Time
  ToWs_Result_Bus_Sig1 : ToWorkspace  VariableName=sig_result_001_001  SaveFormat=Structure With Time
  ToWs_Result_Bus_Sig2 : ToWorkspace  VariableName=sig_result_001_002  SaveFormat=Structure With Time
  ToWs_Result_Bus_Sig3 : ToWorkspace  VariableName=sig_result_001_003  SaveFormat=Structure With Time
  ToWs_Result_Bus_Sig4 : ToWorkspace  VariableName=sig_result_001_004  SaveFormat=Structure With Time
  ToWs_Result_Bus_Sig5 : ToWorkspace  VariableName=sig_result_001_005  SaveFormat=Structure With Time
  ToWs_Result_Bus_Sig6 : ToWorkspace  VariableName=sig_result_001_006  SaveFormat=Structure With Time
  ToWs_Result_Bus_Sig7 : ToWorkspace  VariableName=sig_result_001_007  SaveFormat=Structure With Time
  ToWs_Result_Bus_Sig8 : ToWorkspace  VariableName=sig_result_001_008  SaveFormat=Structure With Time
  ToWs_Result_Bus_Sig9 : ToWorkspace  VariableName=sig_result_001_009  SaveFormat=Structure With Time
  specifyOutputs : Subsystem
  result : Outport
  wires:
  sig_Req_Bus/1 -> BS/1, specifyOutputs/1(sig_Req_Bus)
  BS/1 -> ToWs_Req_Bus_Sig1/1  "<testSig_AccPed_stBrkDes>"
  BS/2 -> ToWs_Req_Bus_Sig2/1  "<testSig_APP_r>"
  BS/3 -> ToWs_Req_Bus_Sig3/1  "<testSig_Brk_st>"
  BS/4 -> ToWs_Req_Bus_Sig4/1  "<testSig_Clth_st>"
  BS/5 -> ToWs_Req_Bus_Sig5/1  "<testSig_CoEng_st>"
  BS/6 -> ToWs_Req_Bus_Sig6/1  "<testSig_CoEng_stEngStop>"
  BS/7 -> ToWs_Req_Bus_Sig7/1  "<testSig_CoETS_stInrDesBrk>"
  BS/8 -> ToWs_Req_Bus_Sig8/1  "<testSig_CoVeh_trqAcs>"
  BS/9 -> ToWs_Req_Bus_Sig9/1  "<testSig_CrCtl_rTraV2NBeg>"
  BS/10 -> ToWs_Req_Bus_Sig10/1  "<testSig_CrCtl_st_raw>"
  BS/11 -> ToWs_Req_Bus_Sig11/1  "<testSig_CrCtl_stOpFunc>"
  BS/12 -> ToWs_Req_Bus_Sig12/1  "<testSig_CrCtl_stStTrans>"
  BS/13 -> ToWs_Req_Bus_Sig13/1  "<testSig_CrCtl_stSub_raw>"
  BS/14 -> ToWs_Req_Bus_Sig14/1  "<testSig_CrCtl_trqReq>"
  BS/15 -> ToWs_Req_Bus_Sig15/1  "<testSig_CrCtl_vDes>"
  BS/16 -> ToWs_Req_Bus_Sig16/1  "<testSig_CrCUI_stBttn>"
  BS/17 -> ToWs_Req_Bus_Sig17/1  "<testSig_EBrk_stPreSelMode>"
  BS/18 -> ToWs_Req_Bus_Sig18/1  "<testSig_Epm_nEng>"
  BS/19 -> ToWs_Req_Bus_Sig19/1  "<testSig_Gbx_bGearShftActv>"
  BS/20 -> ToWs_Req_Bus_Sig20/1  "<testSig_GlbDa_aXFlt>"
  BS/21 -> ToWs_Req_Bus_Sig21/1  "<testSig_GlbDa_stTrqDem>"
  BS/22 -> ToWs_Req_Bus_Sig22/1  "<testSig_GlbDa_vXFlt>"
  BS/23 -> ToWs_Req_Bus_Sig23/1  "<testSig_HndBrk_stDebVal>"
  BS/24 -> ToWs_Req_Bus_Sig24/1  "<testSig_LLim_stCrCtlShOff>"
  BS/25 -> ToWs_Req_Bus_Sig25/1  "<testSig_PT_rTraV2N>"
  BS/26 -> ToWs_Req_Bus_Sig26/1  "<testSig_PT_rTrq>"
  BS/27 -> ToWs_Req_Bus_Sig27/1  "<testSig_PT_trqLos>"
  BS/28 -> ToWs_Req_Bus_Sig28/1  "<testSig_PT_trqWhlMinEng>"
  BS/29 -> ToWs_Req_Bus_Sig29/1  "<testSig_RngMod_trqCrSMin>"
  BS/30 -> ToWs_Req_Bus_Sig30/1  "<testSig_SpdGov_st>"
  BS/31 -> ToWs_Req_Bus_Sig31/1  "<testSig_SpdGov_trqSet>"
  BS/32 -> ToWs_Req_Bus_Sig32/1  "<testSig_T15_st>"
  BS/33 -> ToWs_Req_Bus_Sig33/1  "<testSig_Tra_numGear>"
  BS/34 -> ToWs_Req_Bus_Sig34/1  "<testSig_VehMot_rTrqDfftl>"
  BS/35 -> ToWs_Req_Bus_Sig35/1  "<testSig_WESDem_stCrCtlShutOff>"
  BS/36 -> ToWs_Req_Bus_Sig36/1  "<testSig_CoETS_stTSEATrqSpdReq>"
  BS/37 -> ToWs_Req_Bus_Sig37/1  "<testSig_DSM_bCUT>"
  BS/38 -> ToWs_Req_Bus_Sig38/1  "<testSig_DSM_bTIMECNSTRMP>"
  BS/39 -> ToWs_Req_Bus_Sig39/1  "<testSig_DSM_bSLPCNSTRMP>"
  BS/40 -> ToWs_Req_Bus_Sig40/1  "<testSig_CrCtl_stLck>"
  BS/41 -> ToWs_Req_Bus_Sig41/1  "<testSig_CrCtl_vDesAct>"
  BS/42 -> ToWs_Req_Bus_Sig42/1  "<testSig_CrCtl_rTraV2NSusp>"
  BS/43 -> ToWs_Req_Bus_Sig43/1  "<testSig_CrCtl_stLck_raw>"
  BS/44 -> ToWs_Req_Bus_Sig44/1  "<testSig_CrCtl_stShOff>"
  BS/45 -> ToWs_Req_Bus_Sig45/1  "<testSig_CrCtl_stSuspAct>"
  BS/46 -> ToWs_Req_Bus_Sig46/1  "<testSig_CrCtl_st_raw1>"
  BS/47 -> ToWs_Req_Bus_Sig47/1  "<testSig_CrCtl_stSub_raw1>"
  BS/48 -> ToWs_Req_Bus_Sig48/1  "<testSig_CrCtl_stShOffConStore_mp>"
  BS/49 -> ToWs_Req_Bus_Sig49/1  "<testSig_CrCtl_vDes_raw>"
  BS/50 -> ToWs_Req_Bus_Sig50/1  "<testSig_CrCtl_vDesAct_raw>"
  sig_Result_Bus/1 -> BS_Result/1, specifyOutputs/2(sig_Result_Bus)
  BS_Result/1 -> ToWs_Result_Bus_Sig1/1  "<CrCtl_rTraV2NSusp>"
  BS_Result/2 -> ToWs_Result_Bus_Sig2/1  "<CrCtl_stLck_raw>"
  BS_Result/3 -> ToWs_Result_Bus_Sig3/1  "<CrCtl_stShOff>"
  BS_Result/4 -> ToWs_Result_Bus_Sig4/1  "<CrCtl_stSuspAct>"
  BS_Result/5 -> ToWs_Result_Bus_Sig5/1  "<CrCtl_st_raw1>"
  BS_Result/6 -> ToWs_Result_Bus_Sig6/1  "<CrCtl_stSub_raw1>"
  BS_Result/7 -> ToWs_Result_Bus_Sig7/1  "<CrCtl_stShOffConStore_mp>"
  BS_Result/8 -> ToWs_Result_Bus_Sig8/1  "<CrCtl_vDes_raw>"
  BS_Result/9 -> ToWs_Result_Bus_Sig9/1  "<CrCtl_vDesAct_raw>"
  specifyOutputs/1(result) -> result/1

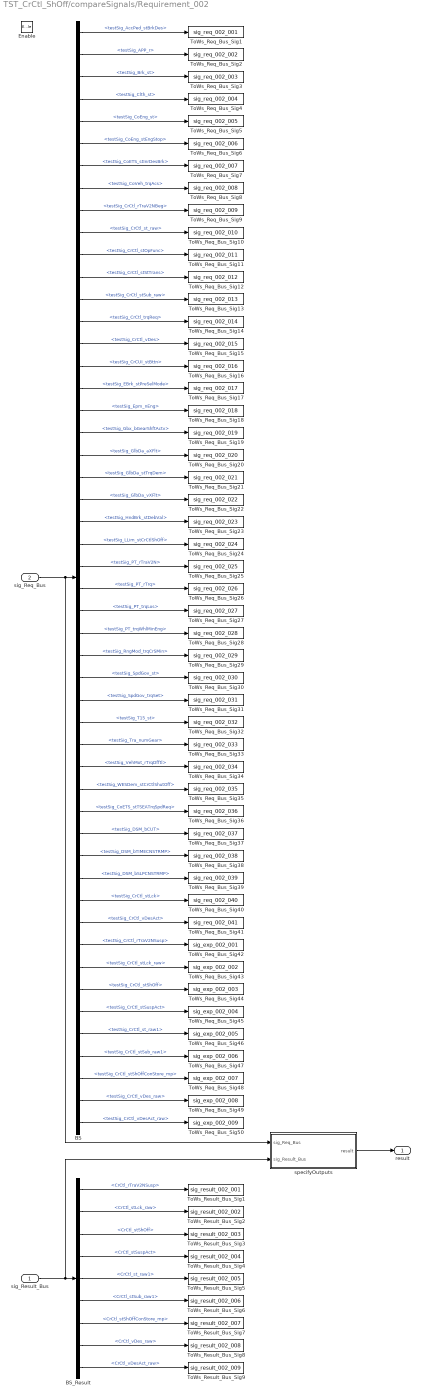
== system TST_CrCtl_ShOff/compareSignals/Requirement_002 ==
  sig_Result_Bus : Inport
  sig_Req_Bus : Inport  Port=2
  Enable : EnablePort
  BS : BusSelector  OutputSignals=testSig_AccPed_stBrkDes,testSig_APP_r,testSig_Brk_st,testSig_Clth_st,testSig_CoEng_st,testSig_CoEng_stEngStop,testSig_CoETS_stInrDesBrk,testSig_CoVeh_trqAcs,testSig_CrCtl_rTraV2NBeg,testSig_CrCtl_st_raw,testSig_CrCtl_stOpFunc,testSig_CrCtl_stStTrans,testSig_CrCtl_stSub_raw,testSig_CrCtl_trqReq,testSig_CrCtl_vDes,testSig_CrCUI_stBttn,testSig_EBrk_stPreSelMode,testSig_Epm_nEng,testSig_Gbx_bGearShftActv,testSig_GlbDa_aXFlt,testSig_GlbDa_stTrqDem,testSig_GlbDa_vXFlt,testSig_HndBrk_stDebVal,testSig_LLim_stCrCtlShOff,testSig_PT_rTraV2N,testSig_PT_rTrq,testSig_PT_trqLos,testSig_PT_trqWhlMinEng,testSig_RngMod_trqCrSMin,testSig_SpdGov_st,testSig_SpdGov_trqSet,testSig_T15_st,testSig_Tra_numGear,testSig_VehMot_rTrqDfftl,testSig_WESDem_stCrCtlShutOff,testSig_CoETS_stTSEATrqSpdReq,testSig_DSM_bCUT,testSig_DSM_bTIMECNSTRMP,testSig_DSM_bSLPCNSTRMP,testSig_CrCtl_stLck,testSig_CrCtl_vDesAct,testSig_CrCtl_rTraV2NSusp,testSig_CrCtl_stLck_raw,testSig_CrCtl_stShOff,testSig_CrCtl_stSuspAct,testSig_CrCtl_st_raw1,testSig_CrCtl_stSub_raw1,testSig_CrCtl_stShOffConStore_mp,testSig_CrCtl_vDes_raw,testSig_CrCtl_vDesAct_raw
  BS_Result : BusSelector  OutputSignals=CrCtl_rTraV2NSusp,CrCtl_stLck_raw,CrCtl_stShOff,CrCtl_stSuspAct,CrCtl_st_raw1,CrCtl_stSub_raw1,CrCtl_stShOffConStore_mp,CrCtl_vDes_raw,CrCtl_vDesAct_raw
  ToWs_Req_Bus_Sig1 : ToWorkspace  VariableName=sig_req_002_001  SaveFormat=Structure With Time
  ToWs_Req_Bus_Sig10 : ToWorkspace  VariableName=sig_req_002_010  SaveFormat=Structure With Time
  ToWs_Req_Bus_Sig11 : ToWorkspace  VariableName=sig_req_002_011  SaveFormat=Structure With Time
  ToWs_Req_Bus_Sig12 : ToWorkspace  VariableName=sig_req_002_012  SaveFormat=Structure With Time
  ToWs_Req_Bus_Sig13 : ToWorkspace  VariableName=sig_req_002_013  SaveFormat=Structure With Time
  ToWs_Req_Bus_Sig14 : ToWorkspace  VariableName=sig_req_002_014  SaveFormat=Structure With Time
  ToWs_Req_Bus_Sig15 : ToWorkspace  VariableName=sig_req_002_015  SaveFormat=Structure With Time
  ToWs_Req_Bus_Sig16 : ToWorkspace  VariableName=sig_req_002_016  SaveFormat=Structure With Time
  ToWs_Req_Bus_Sig17 : ToWorkspace  VariableName=sig_req_002_017  SaveFormat=Structure With Time
  ToWs_Req_Bus_Sig18 : ToWorkspace  VariableName=sig_req_002_018  SaveFormat=Structure With Time
  ToWs_Req_Bus_Sig19 : ToWorkspace  VariableName=sig_req_002_019  SaveFormat=Structure With Time
  ToWs_Req_Bus_Sig2 : ToWorkspace  VariableName=sig_req_002_002  SaveFormat=Structure With Time
  ToWs_Req_Bus_Sig20 : ToWorkspace  VariableName=sig_req_002_020  SaveFormat=Structure With Time
  ToWs_Req_Bus_Sig21 : ToWorkspace  VariableName=sig_req_002_021  SaveFormat=Structure With Time
  ToWs_Req_Bus_Sig22 : ToWorkspace  VariableName=sig_req_002_022  SaveFormat=Structure With Time
  ToWs_Req_Bus_Sig23 : ToWorkspace  VariableName=sig_req_002_023  SaveFormat=Structure With Time
  ToWs_Req_Bus_Sig24 : ToWorkspace  VariableName=sig_req_002_024  SaveFormat=Structure With Time
  ToWs_Req_Bus_Sig25 : ToWorkspace  VariableName=sig_req_002_025  SaveFormat=Structure With Time
  ToWs_Req_Bus_Sig26 : ToWorkspace  VariableName=sig_req_002_026  SaveFormat=Structure With Time
  ToWs_Req_Bus_Sig27 : ToWorkspace  VariableName=sig_req_002_027  SaveFormat=Structure With Time
  ToWs_Req_Bus_Sig28 : ToWorkspace  VariableName=sig_req_002_028  SaveFormat=Structure With Time
  ToWs_Req_Bus_Sig29 : ToWorkspace  VariableName=sig_req_002_029  SaveFormat=Structure With Time
  ToWs_Req_Bus_Sig3 : ToWorkspace  VariableName=sig_req_002_003  SaveFormat=Structure With Time
  ToWs_Req_Bus_Sig30 : ToWorkspace  VariableName=sig_req_002_030  SaveFormat=Structure With Time
  ToWs_Req_Bus_Sig31 : ToWorkspace  VariableName=sig_req_002_031  SaveFormat=Structure With Time
  ToWs_Req_Bus_Sig32 : ToWorkspace  VariableName=sig_req_002_032  SaveFormat=Structure With Time
  ToWs_Req_Bus_Sig33 : ToWorkspace  VariableName=sig_req_002_033  SaveFormat=Structure With Time
  ToWs_Req_Bus_Sig34 : ToWorkspace  VariableName=sig_req_002_034  SaveFormat=Structure With Time
  ToWs_Req_Bus_Sig35 : ToWorkspace  VariableName=sig_req_002_035  SaveFormat=Structure With Time
  ToWs_Req_Bus_Sig36 : ToWorkspace  VariableName=sig_req_002_036  SaveFormat=Structure With Time
  ToWs_Req_Bus_Sig37 : ToWorkspace  VariableName=sig_req_002_037  SaveFormat=Structure With Time
  ToWs_Req_Bus_Sig38 : ToWorkspace  VariableName=sig_req_002_038  SaveFormat=Structure With Time
  ToWs_Req_Bus_Sig39 : ToWorkspace  VariableName=sig_req_002_039  SaveFormat=Structure With Time
  ToWs_Req_Bus_Sig4 : ToWorkspace  VariableName=sig_req_002_004  SaveFormat=Structure With Time
  ToWs_Req_Bus_Sig40 : ToWorkspace  VariableName=sig_req_002_040  SaveFormat=Structure With Time
  ToWs_Req_Bus_Sig41 : ToWorkspace  VariableName=sig_req_002_041  SaveFormat=Structure With Time
  ToWs_Req_Bus_Sig42 : ToWorkspace  VariableName=sig_exp_002_001  SaveFormat=Structure With Time
  ToWs_Req_Bus_Sig43 : ToWorkspace  VariableName=sig_exp_002_002  SaveFormat=Structure With Time
  ToWs_Req_Bus_Sig44 : ToWorkspace  VariableName=sig_exp_002_003  SaveFormat=Structure With Time
  ToWs_Req_Bus_Sig45 : ToWorkspace  VariableName=sig_exp_002_004  SaveFormat=Structure With Time
  ToWs_Req_Bus_Sig46 : ToWorkspace  VariableName=sig_exp_002_005  SaveFormat=Structure With Time
  ToWs_Req_Bus_Sig47 : ToWorkspace  VariableName=sig_exp_002_006  SaveFormat=Structure With Time
  ToWs_Req_Bus_Sig48 : ToWorkspace  VariableName=sig_exp_002_007  SaveFormat=Structure With Time
  ToWs_Req_Bus_Sig49 : ToWorkspace  VariableName=sig_exp_002_008  SaveFormat=Structure With Time
  ToWs_Req_Bus_Sig5 : ToWorkspace  VariableName=sig_req_002_005  SaveFormat=Structure With Time
  ToWs_Req_Bus_Sig50 : ToWorkspace  VariableName=sig_exp_002_009  SaveFormat=Structure With Time
  ToWs_Req_Bus_Sig6 : ToWorkspace  VariableName=sig_req_002_006  SaveFormat=Structure With Time
  ToWs_Req_Bus_Sig7 : ToWorkspace  VariableName=sig_req_002_007  SaveFormat=Structure With Time
  ToWs_Req_Bus_Sig8 : ToWorkspace  VariableName=sig_req_002_008  SaveFormat=Structure With Time
  ToWs_Req_Bus_Sig9 : ToWorkspace  VariableName=sig_req_002_009  SaveFormat=Structure With Time
  ToWs_Result_Bus_Sig1 : ToWorkspace  VariableName=sig_result_002_001  SaveFormat=Structure With Time
  ToWs_Result_Bus_Sig2 : ToWorkspace  VariableName=sig_result_002_002  SaveFormat=Structure With Time
  ToWs_Result_Bus_Sig3 : ToWorkspace  VariableName=sig_result_002_003  SaveFormat=Structure With Time
  ToWs_Result_Bus_Sig4 : ToWorkspace  VariableName=sig_result_002_004  SaveFormat=Structure With Time
  ToWs_Result_Bus_Sig5 : ToWorkspace  VariableName=sig_result_002_005  SaveFormat=Structure With Time
  ToWs_Result_Bus_Sig6 : ToWorkspace  VariableName=sig_result_002_006  SaveFormat=Structure With Time
  ToWs_Result_Bus_Sig7 : ToWorkspace  VariableName=sig_result_002_007  SaveFormat=Structure With Time
  ToWs_Result_Bus_Sig8 : ToWorkspace  VariableName=sig_result_002_008  SaveFormat=Structure With Time
  ToWs_Result_Bus_Sig9 : ToWorkspace  VariableName=sig_result_002_009  SaveFormat=Structure With Time
  specifyOutputs : Subsystem
  result : Outport
  wires:
  sig_Req_Bus/1 -> BS/1, specifyOutputs/1(sig_Req_Bus)
  BS/1 -> ToWs_Req_Bus_Sig1/1  "<testSig_AccPed_stBrkDes>"
  BS/2 -> ToWs_Req_Bus_Sig2/1  "<testSig_APP_r>"
  BS/3 -> ToWs_Req_Bus_Sig3/1  "<testSig_Brk_st>"
  BS/4 -> ToWs_Req_Bus_Sig4/1  "<testSig_Clth_st>"
  BS/5 -> ToWs_Req_Bus_Sig5/1  "<testSig_CoEng_st>"
  BS/6 -> ToWs_Req_Bus_Sig6/1  "<testSig_CoEng_stEngStop>"
  BS/7 -> ToWs_Req_Bus_Sig7/1  "<testSig_CoETS_stInrDesBrk>"
  BS/8 -> ToWs_Req_Bus_Sig8/1  "<testSig_CoVeh_trqAcs>"
  BS/9 -> ToWs_Req_Bus_Sig9/1  "<testSig_CrCtl_rTraV2NBeg>"
  BS/10 -> ToWs_Req_Bus_Sig10/1  "<testSig_CrCtl_st_raw>"
  BS/11 -> ToWs_Req_Bus_Sig11/1  "<testSig_CrCtl_stOpFunc>"
  BS/12 -> ToWs_Req_Bus_Sig12/1  "<testSig_CrCtl_stStTrans>"
  BS/13 -> ToWs_Req_Bus_Sig13/1  "<testSig_CrCtl_stSub_raw>"
  BS/14 -> ToWs_Req_Bus_Sig14/1  "<testSig_CrCtl_trqReq>"
  BS/15 -> ToWs_Req_Bus_Sig15/1  "<testSig_CrCtl_vDes>"
  BS/16 -> ToWs_Req_Bus_Sig16/1  "<testSig_CrCUI_stBttn>"
  BS/17 -> ToWs_Req_Bus_Sig17/1  "<testSig_EBrk_stPreSelMode>"
  BS/18 -> ToWs_Req_Bus_Sig18/1  "<testSig_Epm_nEng>"
  BS/19 -> ToWs_Req_Bus_Sig19/1  "<testSig_Gbx_bGearShftActv>"
  BS/20 -> ToWs_Req_Bus_Sig20/1  "<testSig_GlbDa_aXFlt>"
  BS/21 -> ToWs_Req_Bus_Sig21/1  "<testSig_GlbDa_stTrqDem>"
  BS/22 -> ToWs_Req_Bus_Sig22/1  "<testSig_GlbDa_vXFlt>"
  BS/23 -> ToWs_Req_Bus_Sig23/1  "<testSig_HndBrk_stDebVal>"
  BS/24 -> ToWs_Req_Bus_Sig24/1  "<testSig_LLim_stCrCtlShOff>"
  BS/25 -> ToWs_Req_Bus_Sig25/1  "<testSig_PT_rTraV2N>"
  BS/26 -> ToWs_Req_Bus_Sig26/1  "<testSig_PT_rTrq>"
  BS/27 -> ToWs_Req_Bus_Sig27/1  "<testSig_PT_trqLos>"
  BS/28 -> ToWs_Req_Bus_Sig28/1  "<testSig_PT_trqWhlMinEng>"
  BS/29 -> ToWs_Req_Bus_Sig29/1  "<testSig_RngMod_trqCrSMin>"
  BS/30 -> ToWs_Req_Bus_Sig30/1  "<testSig_SpdGov_st>"
  BS/31 -> ToWs_Req_Bus_Sig31/1  "<testSig_SpdGov_trqSet>"
  BS/32 -> ToWs_Req_Bus_Sig32/1  "<testSig_T15_st>"
  BS/33 -> ToWs_Req_Bus_Sig33/1  "<testSig_Tra_numGear>"
  BS/34 -> ToWs_Req_Bus_Sig34/1  "<testSig_VehMot_rTrqDfftl>"
  BS/35 -> ToWs_Req_Bus_Sig35/1  "<testSig_WESDem_stCrCtlShutOff>"
  BS/36 -> ToWs_Req_Bus_Sig36/1  "<testSig_CoETS_stTSEATrqSpdReq>"
  BS/37 -> ToWs_Req_Bus_Sig37/1  "<testSig_DSM_bCUT>"
  BS/38 -> ToWs_Req_Bus_Sig38/1  "<testSig_DSM_bTIMECNSTRMP>"
  BS/39 -> ToWs_Req_Bus_Sig39/1  "<testSig_DSM_bSLPCNSTRMP>"
  BS/40 -> ToWs_Req_Bus_Sig40/1  "<testSig_CrCtl_stLck>"
  BS/41 -> ToWs_Req_Bus_Sig41/1  "<testSig_CrCtl_vDesAct>"
  BS/42 -> ToWs_Req_Bus_Sig42/1  "<testSig_CrCtl_rTraV2NSusp>"
  BS/43 -> ToWs_Req_Bus_Sig43/1  "<testSig_CrCtl_stLck_raw>"
  BS/44 -> ToWs_Req_Bus_Sig44/1  "<testSig_CrCtl_stShOff>"
  BS/45 -> ToWs_Req_Bus_Sig45/1  "<testSig_CrCtl_stSuspAct>"
  BS/46 -> ToWs_Req_Bus_Sig46/1  "<testSig_CrCtl_st_raw1>"
  BS/47 -> ToWs_Req_Bus_Sig47/1  "<testSig_CrCtl_stSub_raw1>"
  BS/48 -> ToWs_Req_Bus_Sig48/1  "<testSig_CrCtl_stShOffConStore_mp>"
  BS/49 -> ToWs_Req_Bus_Sig49/1  "<testSig_CrCtl_vDes_raw>"
  BS/50 -> ToWs_Req_Bus_Sig50/1  "<testSig_CrCtl_vDesAct_raw>"
  sig_Result_Bus/1 -> BS_Result/1, specifyOutputs/2(sig_Result_Bus)
  BS_Result/1 -> ToWs_Result_Bus_Sig1/1  "<CrCtl_rTraV2NSusp>"
  BS_Result/2 -> ToWs_Result_Bus_Sig2/1  "<CrCtl_stLck_raw>"
  BS_Result/3 -> ToWs_Result_Bus_Sig3/1  "<CrCtl_stShOff>"
  BS_Result/4 -> ToWs_Result_Bus_Sig4/1  "<CrCtl_stSuspAct>"
  BS_Result/5 -> ToWs_Result_Bus_Sig5/1  "<CrCtl_st_raw1>"
  BS_Result/6 -> ToWs_Result_Bus_Sig6/1  "<CrCtl_stSub_raw1>"
  BS_Result/7 -> ToWs_Result_Bus_Sig7/1  "<CrCtl_stShOffConStore_mp>"
  BS_Result/8 -> ToWs_Result_Bus_Sig8/1  "<CrCtl_vDes_raw>"
  BS_Result/9 -> ToWs_Result_Bus_Sig9/1  "<CrCtl_vDesAct_raw>"
  specifyOutputs/1(result) -> result/1

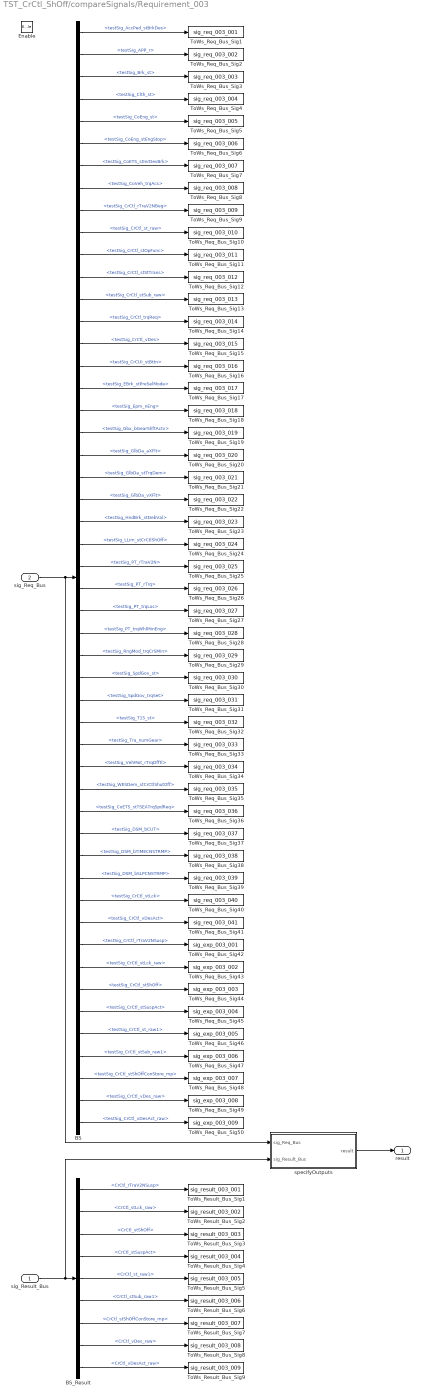
== system TST_CrCtl_ShOff/compareSignals/Requirement_003 ==
  sig_Result_Bus : Inport
  sig_Req_Bus : Inport  Port=2
  Enable : EnablePort
  BS : BusSelector  OutputSignals=testSig_AccPed_stBrkDes,testSig_APP_r,testSig_Brk_st,testSig_Clth_st,testSig_CoEng_st,testSig_CoEng_stEngStop,testSig_CoETS_stInrDesBrk,testSig_CoVeh_trqAcs,testSig_CrCtl_rTraV2NBeg,testSig_CrCtl_st_raw,testSig_CrCtl_stOpFunc,testSig_CrCtl_stStTrans,testSig_CrCtl_stSub_raw,testSig_CrCtl_trqReq,testSig_CrCtl_vDes,testSig_CrCUI_stBttn,testSig_EBrk_stPreSelMode,testSig_Epm_nEng,testSig_Gbx_bGearShftActv,testSig_GlbDa_aXFlt,testSig_GlbDa_stTrqDem,testSig_GlbDa_vXFlt,testSig_HndBrk_stDebVal,testSig_LLim_stCrCtlShOff,testSig_PT_rTraV2N,testSig_PT_rTrq,testSig_PT_trqLos,testSig_PT_trqWhlMinEng,testSig_RngMod_trqCrSMin,testSig_SpdGov_st,testSig_SpdGov_trqSet,testSig_T15_st,testSig_Tra_numGear,testSig_VehMot_rTrqDfftl,testSig_WESDem_stCrCtlShutOff,testSig_CoETS_stTSEATrqSpdReq,testSig_DSM_bCUT,testSig_DSM_bTIMECNSTRMP,testSig_DSM_bSLPCNSTRMP,testSig_CrCtl_stLck,testSig_CrCtl_vDesAct,testSig_CrCtl_rTraV2NSusp,testSig_CrCtl_stLck_raw,testSig_CrCtl_stShOff,testSig_CrCtl_stSuspAct,testSig_CrCtl_st_raw1,testSig_CrCtl_stSub_raw1,testSig_CrCtl_stShOffConStore_mp,testSig_CrCtl_vDes_raw,testSig_CrCtl_vDesAct_raw
  BS_Result : BusSelector  OutputSignals=CrCtl_rTraV2NSusp,CrCtl_stLck_raw,CrCtl_stShOff,CrCtl_stSuspAct,CrCtl_st_raw1,CrCtl_stSub_raw1,CrCtl_stShOffConStore_mp,CrCtl_vDes_raw,CrCtl_vDesAct_raw
  ToWs_Req_Bus_Sig1 : ToWorkspace  VariableName=sig_req_003_001  SaveFormat=Structure With Time
  ToWs_Req_Bus_Sig10 : ToWorkspace  VariableName=sig_req_003_010  SaveFormat=Structure With Time
  ToWs_Req_Bus_Sig11 : ToWorkspace  VariableName=sig_req_003_011  SaveFormat=Structure With Time
  ToWs_Req_Bus_Sig12 : ToWorkspace  VariableName=sig_req_003_012  SaveFormat=Structure With Time
  ToWs_Req_Bus_Sig13 : ToWorkspace  VariableName=sig_req_003_013  SaveFormat=Structure With Time
  ToWs_Req_Bus_Sig14 : ToWorkspace  VariableName=sig_req_003_014  SaveFormat=Structure With Time
  ToWs_Req_Bus_Sig15 : ToWorkspace  VariableName=sig_req_003_015  SaveFormat=Structure With Time
  ToWs_Req_Bus_Sig16 : ToWorkspace  VariableName=sig_req_003_016  SaveFormat=Structure With Time
  ToWs_Req_Bus_Sig17 : ToWorkspace  VariableName=sig_req_003_017  SaveFormat=Structure With Time
  ToWs_Req_Bus_Sig18 : ToWorkspace  VariableName=sig_req_003_018  SaveFormat=Structure With Time
  ToWs_Req_Bus_Sig19 : ToWorkspace  VariableName=sig_req_003_019  SaveFormat=Structure With Time
  ToWs_Req_Bus_Sig2 : ToWorkspace  VariableName=sig_req_003_002  SaveFormat=Structure With Time
  ToWs_Req_Bus_Sig20 : ToWorkspace  VariableName=sig_req_003_020  SaveFormat=Structure With Time
  ToWs_Req_Bus_Sig21 : ToWorkspace  VariableName=sig_req_003_021  SaveFormat=Structure With Time
  ToWs_Req_Bus_Sig22 : ToWorkspace  VariableName=sig_req_003_022  SaveFormat=Structure With Time
  ToWs_Req_Bus_Sig23 : ToWorkspace  VariableName=sig_req_003_023  SaveFormat=Structure With Time
  ToWs_Req_Bus_Sig24 : ToWorkspace  VariableName=sig_req_003_024  SaveFormat=Structure With Time
  ToWs_Req_Bus_Sig25 : ToWorkspace  VariableName=sig_req_003_025  SaveFormat=Structure With Time
  ToWs_Req_Bus_Sig26 : ToWorkspace  VariableName=sig_req_003_026  SaveFormat=Structure With Time
  ToWs_Req_Bus_Sig27 : ToWorkspace  VariableName=sig_req_003_027  SaveFormat=Structure With Time
  ToWs_Req_Bus_Sig28 : ToWorkspace  VariableName=sig_req_003_028  SaveFormat=Structure With Time
  ToWs_Req_Bus_Sig29 : ToWorkspace  VariableName=sig_req_003_029  SaveFormat=Structure With Time
  ToWs_Req_Bus_Sig3 : ToWorkspace  VariableName=sig_req_003_003  SaveFormat=Structure With Time
  ToWs_Req_Bus_Sig30 : ToWorkspace  VariableName=sig_req_003_030  SaveFormat=Structure With Time
  ToWs_Req_Bus_Sig31 : ToWorkspace  VariableName=sig_req_003_031  SaveFormat=Structure With Time
  ToWs_Req_Bus_Sig32 : ToWorkspace  VariableName=sig_req_003_032  SaveFormat=Structure With Time
  ToWs_Req_Bus_Sig33 : ToWorkspace  VariableName=sig_req_003_033  SaveFormat=Structure With Time
  ToWs_Req_Bus_Sig34 : ToWorkspace  VariableName=sig_req_003_034  SaveFormat=Structure With Time
  ToWs_Req_Bus_Sig35 : ToWorkspace  VariableName=sig_req_003_035  SaveFormat=Structure With Time
  ToWs_Req_Bus_Sig36 : ToWorkspace  VariableName=sig_req_003_036  SaveFormat=Structure With Time
  ToWs_Req_Bus_Sig37 : ToWorkspace  VariableName=sig_req_003_037  SaveFormat=Structure With Time
  ToWs_Req_Bus_Sig38 : ToWorkspace  VariableName=sig_req_003_038  SaveFormat=Structure With Time
  ToWs_Req_Bus_Sig39 : ToWorkspace  VariableName=sig_req_003_039  SaveFormat=Structure With Time
  ToWs_Req_Bus_Sig4 : ToWorkspace  VariableName=sig_req_003_004  SaveFormat=Structure With Time
  ToWs_Req_Bus_Sig40 : ToWorkspace  VariableName=sig_req_003_040  SaveFormat=Structure With Time
  ToWs_Req_Bus_Sig41 : ToWorkspace  VariableName=sig_req_003_041  SaveFormat=Structure With Time
  ToWs_Req_Bus_Sig42 : ToWorkspace  VariableName=sig_exp_003_001  SaveFormat=Structure With Time
  ToWs_Req_Bus_Sig43 : ToWorkspace  VariableName=sig_exp_003_002  SaveFormat=Structure With Time
  ToWs_Req_Bus_Sig44 : ToWorkspace  VariableName=sig_exp_003_003  SaveFormat=Structure With Time
  ToWs_Req_Bus_Sig45 : ToWorkspace  VariableName=sig_exp_003_004  SaveFormat=Structure With Time
  ToWs_Req_Bus_Sig46 : ToWorkspace  VariableName=sig_exp_003_005  SaveFormat=Structure With Time
  ToWs_Req_Bus_Sig47 : ToWorkspace  VariableName=sig_exp_003_006  SaveFormat=Structure With Time
  ToWs_Req_Bus_Sig48 : ToWorkspace  VariableName=sig_exp_003_007  SaveFormat=Structure With Time
  ToWs_Req_Bus_Sig49 : ToWorkspace  VariableName=sig_exp_003_008  SaveFormat=Structure With Time
  ToWs_Req_Bus_Sig5 : ToWorkspace  VariableName=sig_req_003_005  SaveFormat=Structure With Time
  ToWs_Req_Bus_Sig50 : ToWorkspace  VariableName=sig_exp_003_009  SaveFormat=Structure With Time
  ToWs_Req_Bus_Sig6 : ToWorkspace  VariableName=sig_req_003_006  SaveFormat=Structure With Time
  ToWs_Req_Bus_Sig7 : ToWorkspace  VariableName=sig_req_003_007  SaveFormat=Structure With Time
  ToWs_Req_Bus_Sig8 : ToWorkspace  VariableName=sig_req_003_008  SaveFormat=Structure With Time
  ToWs_Req_Bus_Sig9 : ToWorkspace  VariableName=sig_req_003_009  SaveFormat=Structure With Time
  ToWs_Result_Bus_Sig1 : ToWorkspace  VariableName=sig_result_003_001  SaveFormat=Structure With Time
  ToWs_Result_Bus_Sig2 : ToWorkspace  VariableName=sig_result_003_002  SaveFormat=Structure With Time
  ToWs_Result_Bus_Sig3 : ToWorkspace  VariableName=sig_result_003_003  SaveFormat=Structure With Time
  ToWs_Result_Bus_Sig4 : ToWorkspace  VariableName=sig_result_003_004  SaveFormat=Structure With Time
  ToWs_Result_Bus_Sig5 : ToWorkspace  VariableName=sig_result_003_005  SaveFormat=Structure With Time
  ToWs_Result_Bus_Sig6 : ToWorkspace  VariableName=sig_result_003_006  SaveFormat=Structure With Time
  ToWs_Result_Bus_Sig7 : ToWorkspace  VariableName=sig_result_003_007  SaveFormat=Structure With Time
  ToWs_Result_Bus_Sig8 : ToWorkspace  VariableName=sig_result_003_008  SaveFormat=Structure With Time
  ToWs_Result_Bus_Sig9 : ToWorkspace  VariableName=sig_result_003_009  SaveFormat=Structure With Time
  specifyOutputs : Subsystem
  result : Outport
  wires:
  sig_Req_Bus/1 -> BS/1, specifyOutputs/1(sig_Req_Bus)
  BS/1 -> ToWs_Req_Bus_Sig1/1  "<testSig_AccPed_stBrkDes>"
  BS/2 -> ToWs_Req_Bus_Sig2/1  "<testSig_APP_r>"
  BS/3 -> ToWs_Req_Bus_Sig3/1  "<testSig_Brk_st>"
  BS/4 -> ToWs_Req_Bus_Sig4/1  "<testSig_Clth_st>"
  BS/5 -> ToWs_Req_Bus_Sig5/1  "<testSig_CoEng_st>"
  BS/6 -> ToWs_Req_Bus_Sig6/1  "<testSig_CoEng_stEngStop>"
  BS/7 -> ToWs_Req_Bus_Sig7/1  "<testSig_CoETS_stInrDesBrk>"
  BS/8 -> ToWs_Req_Bus_Sig8/1  "<testSig_CoVeh_trqAcs>"
  BS/9 -> ToWs_Req_Bus_Sig9/1  "<testSig_CrCtl_rTraV2NBeg>"
  BS/10 -> ToWs_Req_Bus_Sig10/1  "<testSig_CrCtl_st_raw>"
  BS/11 -> ToWs_Req_Bus_Sig11/1  "<testSig_CrCtl_stOpFunc>"
  BS/12 -> ToWs_Req_Bus_Sig12/1  "<testSig_CrCtl_stStTrans>"
  BS/13 -> ToWs_Req_Bus_Sig13/1  "<testSig_CrCtl_stSub_raw>"
  BS/14 -> ToWs_Req_Bus_Sig14/1  "<testSig_CrCtl_trqReq>"
  BS/15 -> ToWs_Req_Bus_Sig15/1  "<testSig_CrCtl_vDes>"
  BS/16 -> ToWs_Req_Bus_Sig16/1  "<testSig_CrCUI_stBttn>"
  BS/17 -> ToWs_Req_Bus_Sig17/1  "<testSig_EBrk_stPreSelMode>"
  BS/18 -> ToWs_Req_Bus_Sig18/1  "<testSig_Epm_nEng>"
  BS/19 -> ToWs_Req_Bus_Sig19/1  "<testSig_Gbx_bGearShftActv>"
  BS/20 -> ToWs_Req_Bus_Sig20/1  "<testSig_GlbDa_aXFlt>"
  BS/21 -> ToWs_Req_Bus_Sig21/1  "<testSig_GlbDa_stTrqDem>"
  BS/22 -> ToWs_Req_Bus_Sig22/1  "<testSig_GlbDa_vXFlt>"
  BS/23 -> ToWs_Req_Bus_Sig23/1  "<testSig_HndBrk_stDebVal>"
  BS/24 -> ToWs_Req_Bus_Sig24/1  "<testSig_LLim_stCrCtlShOff>"
  BS/25 -> ToWs_Req_Bus_Sig25/1  "<testSig_PT_rTraV2N>"
  BS/26 -> ToWs_Req_Bus_Sig26/1  "<testSig_PT_rTrq>"
  BS/27 -> ToWs_Req_Bus_Sig27/1  "<testSig_PT_trqLos>"
  BS/28 -> ToWs_Req_Bus_Sig28/1  "<testSig_PT_trqWhlMinEng>"
  BS/29 -> ToWs_Req_Bus_Sig29/1  "<testSig_RngMod_trqCrSMin>"
  BS/30 -> ToWs_Req_Bus_Sig30/1  "<testSig_SpdGov_st>"
  BS/31 -> ToWs_Req_Bus_Sig31/1  "<testSig_SpdGov_trqSet>"
  BS/32 -> ToWs_Req_Bus_Sig32/1  "<testSig_T15_st>"
  BS/33 -> ToWs_Req_Bus_Sig33/1  "<testSig_Tra_numGear>"
  BS/34 -> ToWs_Req_Bus_Sig34/1  "<testSig_VehMot_rTrqDfftl>"
  BS/35 -> ToWs_Req_Bus_Sig35/1  "<testSig_WESDem_stCrCtlShutOff>"
  BS/36 -> ToWs_Req_Bus_Sig36/1  "<testSig_CoETS_stTSEATrqSpdReq>"
  BS/37 -> ToWs_Req_Bus_Sig37/1  "<testSig_DSM_bCUT>"
  BS/38 -> ToWs_Req_Bus_Sig38/1  "<testSig_DSM_bTIMECNSTRMP>"
  BS/39 -> ToWs_Req_Bus_Sig39/1  "<testSig_DSM_bSLPCNSTRMP>"
  BS/40 -> ToWs_Req_Bus_Sig40/1  "<testSig_CrCtl_stLck>"
  BS/41 -> ToWs_Req_Bus_Sig41/1  "<testSig_CrCtl_vDesAct>"
  BS/42 -> ToWs_Req_Bus_Sig42/1  "<testSig_CrCtl_rTraV2NSusp>"
  BS/43 -> ToWs_Req_Bus_Sig43/1  "<testSig_CrCtl_stLck_raw>"
  BS/44 -> ToWs_Req_Bus_Sig44/1  "<testSig_CrCtl_stShOff>"
  BS/45 -> ToWs_Req_Bus_Sig45/1  "<testSig_CrCtl_stSuspAct>"
  BS/46 -> ToWs_Req_Bus_Sig46/1  "<testSig_CrCtl_st_raw1>"
  BS/47 -> ToWs_Req_Bus_Sig47/1  "<testSig_CrCtl_stSub_raw1>"
  BS/48 -> ToWs_Req_Bus_Sig48/1  "<testSig_CrCtl_stShOffConStore_mp>"
  BS/49 -> ToWs_Req_Bus_Sig49/1  "<testSig_CrCtl_vDes_raw>"
  BS/50 -> ToWs_Req_Bus_Sig50/1  "<testSig_CrCtl_vDesAct_raw>"
  sig_Result_Bus/1 -> BS_Result/1, specifyOutputs/2(sig_Result_Bus)
  BS_Result/1 -> ToWs_Result_Bus_Sig1/1  "<CrCtl_rTraV2NSusp>"
  BS_Result/2 -> ToWs_Result_Bus_Sig2/1  "<CrCtl_stLck_raw>"
  BS_Result/3 -> ToWs_Result_Bus_Sig3/1  "<CrCtl_stShOff>"
  BS_Result/4 -> ToWs_Result_Bus_Sig4/1  "<CrCtl_stSuspAct>"
  BS_Result/5 -> ToWs_Result_Bus_Sig5/1  "<CrCtl_st_raw1>"
  BS_Result/6 -> ToWs_Result_Bus_Sig6/1  "<CrCtl_stSub_raw1>"
  BS_Result/7 -> ToWs_Result_Bus_Sig7/1  "<CrCtl_stShOffConStore_mp>"
  BS_Result/8 -> ToWs_Result_Bus_Sig8/1  "<CrCtl_vDes_raw>"
  BS_Result/9 -> ToWs_Result_Bus_Sig9/1  "<CrCtl_vDesAct_raw>"
  specifyOutputs/1(result) -> result/1
